simulink model "Lab_1"  (R2025b)
settings: Solver=VariableStepAuto  StartTime=0.0  StopTime=10.0  RelTol=1e-3
undefined symbols (not defined in the file): A, a0, a1, a2, a3, B, C, D
settings Model: Creator=ASUS  LastModifiedBy=ASUS

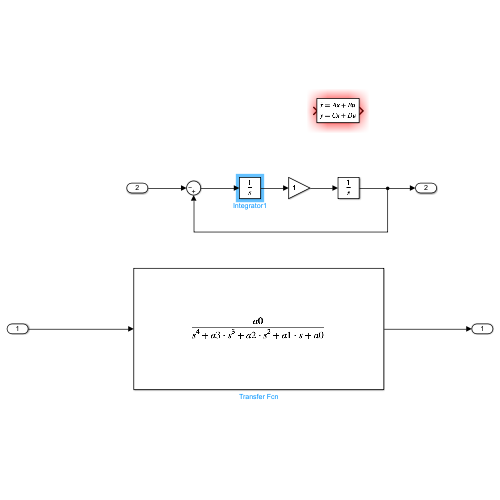
[thumbnail: Simulink's stored preview of the top-level diagram]
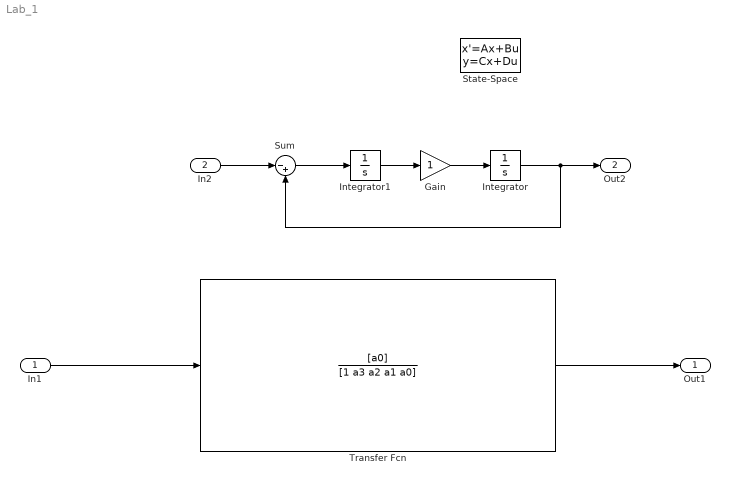
== system Lab_1 ==
  In1 : Inport
  In2 : Inport  Port=2
  Gain : Gain
  Integrator : Integrator
  Integrator1 : Integrator
  State-Space : StateSpace  A=A  B=B  C=C  D=D  InitialCondition=0
  Sum : Sum  Inputs=|-+
  Transfer Fcn : TransferFcn  Numerator=[a0]  Denominator=[1 a3 a2 a1 a0]
  Out1 : Outport
  Out2 : Outport  Port=2
  wires:
  In1/1 -> Transfer Fcn/1
  Transfer Fcn/1 -> Out1/1
  In2/1 -> Sum/1
  Sum/1 -> Integrator1/1
  Integrator1/1 -> Gain/1
  Gain/1 -> Integrator/1
  Integrator/1 -> Sum/2, Out2/1
